simulink model "PI_controller_part1"  (R2019b)
settings: Solver=VariableStepAuto  StartTime=0.0  StopTime=10.0  RelTol=1e-3
values from neighbouring files (symbols this model uses):
  Cs1 = tf([Kc(1)*tauI(1) Kc(1)], [tauI(1) 0])    [PI_controller_part1_params.m]
  Cs2 = tf([Kc(2)*tauI(2) Kc(2)], [tauI(2) 0])    [PI_controller_part1_params.m]
  Cs3 = tf([Kc(3)*tauI(3) Kc(3)], [tauI(3) 0])    [PI_controller_part1_params.m]
  Gs = tf(b, [1 a])    [PI_controller_part1_params.m]
settings Model: Creator=adityaaaap  LastModifiedBy=adityaaaap

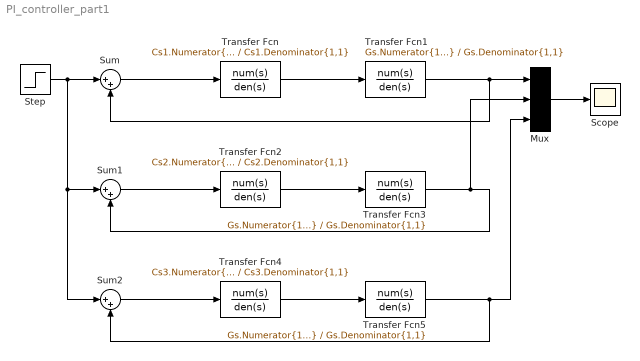
== system PI_controller_part1 ==
  Mux : Mux  Inputs=3
  Scope : Scope
  Step : Step  Time=0  SampleTime=0
  Sum : Sum  Inputs=|++
  Sum1 : Sum  Inputs=|++
  Sum2 : Sum  Inputs=|++
  Transfer Fcn : TransferFcn  Numerator=Cs1.Numerator{1,1}  Denominator=Cs1.Denominator{1,1}
  Transfer Fcn1 : TransferFcn  Numerator=Gs.Numerator{1,1}  Denominator=Gs.Denominator{1,1}
  Transfer Fcn2 : TransferFcn  Numerator=Cs2.Numerator{1,1}  Denominator=Cs2.Denominator{1,1}
  Transfer Fcn3 : TransferFcn  Numerator=Gs.Numerator{1,1}  Denominator=Gs.Denominator{1,1}
  Transfer Fcn4 : TransferFcn  Numerator=Cs3.Numerator{1,1}  Denominator=Cs3.Denominator{1,1}
  Transfer Fcn5 : TransferFcn  Numerator=Gs.Numerator{1,1}  Denominator=Gs.Denominator{1,1}
  wires:
  Step/1 -> Sum2/1, Sum1/1, Sum/1
  Mux/1 -> Scope/1
  Sum/1 -> Transfer Fcn/1
  Transfer Fcn/1 -> Transfer Fcn1/1
  Transfer Fcn1/1 -> Sum/2, Mux/1
  Transfer Fcn2/1 -> Transfer Fcn3/1
  Transfer Fcn3/1 -> Sum1/2, Mux/2
  Sum1/1 -> Transfer Fcn2/1
  Transfer Fcn4/1 -> Transfer Fcn5/1
  Transfer Fcn5/1 -> Mux/3, Sum2/2
  Sum2/1 -> Transfer Fcn4/1
